simulink model "chap04_46"  (R2021a)
settings: Solver=FixedStepDiscrete  StartTime=0.0  StopTime=30  FixedStep=0.001  RelTol=1e-3
undefined symbols (not defined in the file): DiscIntNeverNeededParam
libraries: simulink x4
(part 1 of 4)
settings Model: Creator=陈天兴  LastModifiedBy=陈天兴

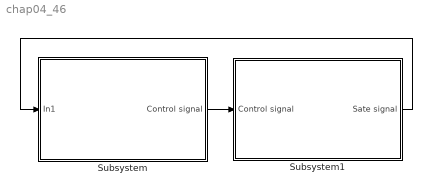
== system chap04_46 ==
  Subsystem : Subsystem
  Subsystem1 : Subsystem
  wires:
  Subsystem/1(Control signal) -> Subsystem1/1(Control signal)
  Subsystem1/1(Sate signal) -> Subsystem/1(In1)

== system chap04_46/Subsystem ==
  In1 : Inport
  Bus Creator : BusCreator  Inputs=6
  Bus Creator2 : BusCreator  Inputs=2
  Subsystem : Subsystem
  Subsystem1 : Subsystem
  Subsystem2 : Subsystem
  Subsystem3 : Subsystem
  Subsystem4 : Subsystem
  Subsystem5 : Subsystem
  Control signal : Outport
  wires:
  Bus Creator2/1 -> Subsystem/1(In19), Subsystem2/1(In19), Subsystem5/1(In19), Subsystem4/1(In19), Subsystem1/1(In19), Subsystem3/1(In19)
  Subsystem5/1(u3) -> Bus Creator/3
  Subsystem3/1(u4) -> Bus Creator/4
  Subsystem1/1(u5) -> Bus Creator/5
  Subsystem/1(u1) -> Bus Creator/1
  Subsystem2/1(u2) -> Bus Creator/2
  Subsystem4/1(u6) -> Bus Creator/6
  Bus Creator/1 -> [control], Control signal/1
  In1/1 -> Bus Creator2/1  "state(t)"
  [control] -> Bus Creator2/2  "control"

== system chap04_46/Subsystem1 ==
  Control signal : Inport
  Bus Creator : BusCreator  Inputs=7
  Bus Creator1 : BusCreator  Inputs=6
  Bus Selector : BusSelector  OutputSignals=node1.ux,node1.uy,node1.uz
  Bus Selector1 : BusSelector  OutputSignals=node2.ux,node2.uy,node2.uz
  Bus Selector2 : BusSelector  OutputSignals=node3.ux,node3.uy,node3.uz
  Bus Selector3 : BusSelector  OutputSignals=node4.ux,node4.uy,node4.uz
  Bus Selector4 : BusSelector  OutputSignals=node5.ux,node5.uy,node5.uz
  Bus Selector5 : BusSelector  OutputSignals=node6.ux,node6.uy,node6.uz
  Constant2 : Constant
  Scope : Scope  NumInputPorts=3
  Subsystem : Subsystem
  Subsystem1 : Subsystem
  Subsystem2 : Subsystem
  Subsystem3 : Subsystem
  Subsystem4 : Subsystem
  Subsystem5 : Subsystem
  Subsystem6 : Subsystem
  Subsystem7 : Subsystem
  Sate signal : Outport
  wires:
  Bus Creator/1 -> Sate signal/1
  Control signal/1 -> Bus Selector/1, Bus Selector1/1, Bus Selector5/1, Bus Selector4/1, Bus Selector3/1, Bus Selector2/1
  Bus Selector/1 -> Subsystem/4(ut1x)  "<ux>"
  Bus Selector/2 -> Subsystem/5(ut1y)  "<uy>"
  Bus Selector/3 -> Subsystem/6(ut1z)  "<uz>"
  Bus Selector1/1 -> Subsystem1/4(ut2x)  "<ux>"
  Bus Selector1/2 -> Subsystem1/5(ut2y)  "<uy>"
  Bus Selector1/3 -> Subsystem1/6(ut2z)  "<uz>"
  Bus Selector2/1 -> Subsystem2/4(ut3x)  "<ux>"
  Bus Selector2/2 -> Subsystem2/5(ut3y)  "<uy>"
  Bus Selector2/3 -> Subsystem2/6(ut3z)  "<uz>"
  Bus Selector3/1 -> Subsystem3/4(ut4x)  "<ux>"
  Bus Selector3/2 -> Subsystem3/5(ut4y)  "<uy>"
  Bus Selector3/3 -> Subsystem3/6(ut4z)  "<uz>"
  Bus Selector4/1 -> Subsystem4/4(ut5x)  "<ux>"
  Bus Selector4/2 -> Subsystem4/5(ut5y)  "<uy>"
  Bus Selector4/3 -> Subsystem4/6(ut5z)  "<uz>"
  Bus Selector5/1 -> Subsystem5/4(ut6x)  "<ux>"
  Bus Selector5/2 -> Subsystem5/5(ut6y)  "<uy>"
  Bus Selector5/3 -> Subsystem5/6(ut6z)  "<uz>"
  Subsystem5/1(node6) -> Bus Creator/7
  Subsystem4/1(node5) -> Bus Creator/6
  Subsystem3/1(node4) -> Bus Creator/5
  Subsystem2/1(node3) -> Bus Creator/4
  Subsystem1/1(node2) -> Bus Creator/3
  Subsystem/1(node1) -> Bus Creator/2
  Subsystem6/5(vy) -> Bus Creator1/5  "vy"
  Subsystem6/2(xy) -> Bus Creator1/2  "xy"
  Subsystem6/3(xz) -> Bus Creator1/3  "xz"
  Subsystem6/4(vx) -> Bus Creator1/4  "vx"
  Subsystem6/6(vz) -> Bus Creator1/6  "vz"
  Bus Creator1/1 -> Bus Creator/1  "node0"
  Subsystem6/1(xx) -> Bus Creator1/1  "xx"
  Subsystem7/2(dy) -> Subsystem/2(dy), Subsystem5/2(dy), Subsystem4/2(dy), Subsystem3/2(dy), Subsystem2/2(dy), Subsystem1/2(dy), Scope/2  "dy"
  Subsystem7/3(dz) -> Subsystem5/3(dz), Subsystem4/3(dz), Subsystem3/3(dz), Subsystem2/3(dz), Subsystem1/3(dz), Subsystem/3(dz), Scope/3  "dz"
  Subsystem7/1(dx) -> Subsystem3/1(dx), Subsystem5/1(dx), Subsystem4/1(dx), Subsystem2/1(dx), Subsystem1/1(dx), Subsystem/1(dx), Scope/1  "dx"
  Constant2/1 -> Subsystem7/1(switch)

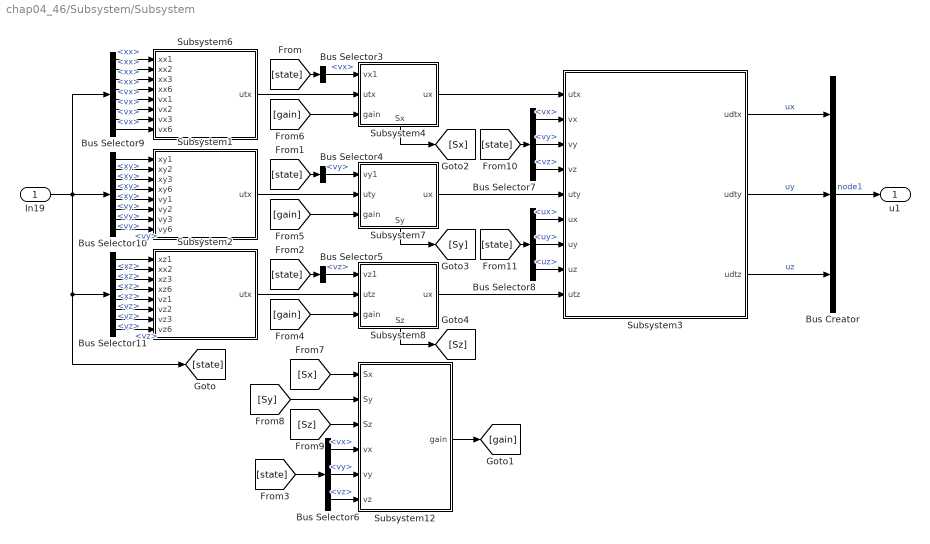
== system chap04_46/Subsystem/Subsystem ==
  In19 : Inport
  Bus Creator : BusCreator  Inputs=3
  Bus Selector10 : BusSelector  OutputSignals=state(t).node1.xy,state(t).node2.xy,state(t).node3.xy,state(t).node6.xy,state(t).node1.vy,state(t).node2.vy,state(t).node3.vy,state(t).node6.vy
  Bus Selector11 : BusSelector  OutputSignals=state(t).node1.xz,state(t).node2.xz,state(t).node3.xz,state(t).node6.xz,state(t).node1.vz,state(t).node2.vz,state(t).node3.vz,state(t).node6.vz
  Bus Selector3 : BusSelector  OutputSignals=state(t).node1.vx
  Bus Selector4 : BusSelector  OutputSignals=state(t).node1.vy
  Bus Selector5 : BusSelector  OutputSignals=state(t).node1.vz
  Bus Selector6 : BusSelector  OutputSignals=state(t).node1.vx,state(t).node1.vy,state(t).node1.vz
  Bus Selector7 : BusSelector  OutputSignals=state(t).node1.vx,state(t).node1.vy,state(t).node1.vz
  Bus Selector8 : BusSelector  OutputSignals=control.node1.ux,control.node1.uy,control.node1.uz
  Bus Selector9 : BusSelector  OutputSignals=state(t).node1.xx,state(t).node2.xx,state(t).node3.xx,state(t).node6.xx,state(t).node1.vx,state(t).node2.vx,state(t).node3.vx,state(t).node6.vx
  Subsystem1 : Subsystem
  Subsystem12 : Subsystem
  Subsystem2 : Subsystem
  Subsystem3 : Subsystem
  Subsystem4 : Subsystem
      settings: PortSchema="{\"entries\":[{\"content\":{\"sides\":[{\"content\":{\"connectorIds\":[\"In1\",\"In2\",\"In3\"]},\"type\":\"ConnectorPlacement.EquallySpacedRectSide\",\"uuid\":\"3c32f130-2df4-4697-80e9-267a8217898e\"},{\"content\":{\"connectorIds\":[\"Out1\"],\"side\":\"RIGHT\"},\"type\":\"ConnectorPlacement.EquallySpacedRectSide\",\"uuid\":\"840675a7-4714-440f-a6ce-75eff1b2763f\"},{\"content\":{\"connectorIds\":[],\"side\":\"TOP\"},\"type\":\"ConnectorPlacement.EquallySpacedRectSide\",\"uuid\":\"5c23af56-4ec3-4a39-a531-12998a0be3c8\"},{\"content\":{\"connectorIds\":[\"Out2\"],\"side\":\"BOTTOM\"},\"type\":\"ConnectorPlacement.EquallySpacedRectSide\",\"uuid\":\"31d953fb-65a0-42e9-a844-060de010f298\"}]},\"type\":\"ConnectorPlacement.EquallySpacedConnector\",\"uuid\":\"61b27aa3-5880-401e-bae3-4611093a191a\"}],\"packageUris\":[\"http://schema.mathworks.com/mf0/Connector/R2020b\"],\"version\":\"1.0\"}"
  Subsystem6 : Subsystem
  Subsystem7 : Subsystem
      settings: PortSchema="{\"entries\":[{\"content\":{\"sides\":[{\"content\":{\"connectorIds\":[\"In1\",\"In2\",\"In3\"]},\"type\":\"ConnectorPlacement.EquallySpacedRectSide\",\"uuid\":\"3c32f130-2df4-4697-80e9-267a8217898e\"},{\"content\":{\"connectorIds\":[\"Out1\"],\"side\":\"RIGHT\"},\"type\":\"ConnectorPlacement.EquallySpacedRectSide\",\"uuid\":\"840675a7-4714-440f-a6ce-75eff1b2763f\"},{\"content\":{\"connectorIds\":[],\"side\":\"TOP\"},\"type\":\"ConnectorPlacement.EquallySpacedRectSide\",\"uuid\":\"5c23af56-4ec3-4a39-a531-12998a0be3c8\"},{\"content\":{\"connectorIds\":[\"Out2\"],\"side\":\"BOTTOM\"},\"type\":\"ConnectorPlacement.EquallySpacedRectSide\",\"uuid\":\"31d953fb-65a0-42e9-a844-060de010f298\"}]},\"type\":\"ConnectorPlacement.EquallySpacedConnector\",\"uuid\":\"61b27aa3-5880-401e-bae3-4611093a191a\"}],\"packageUris\":[\"http://schema.mathworks.com/mf0/Connector/R2020b\"],\"version\":\"1.0\"}"
  Subsystem8 : Subsystem
      settings: PortSchema="{\"entries\":[{\"content\":{\"sides\":[{\"content\":{\"connectorIds\":[\"In1\",\"In2\",\"In3\"]},\"type\":\"ConnectorPlacement.EquallySpacedRectSide\",\"uuid\":\"3c32f130-2df4-4697-80e9-267a8217898e\"},{\"content\":{\"connectorIds\":[\"Out1\"],\"side\":\"RIGHT\"},\"type\":\"ConnectorPlacement.EquallySpacedRectSide\",\"uuid\":\"840675a7-4714-440f-a6ce-75eff1b2763f\"},{\"content\":{\"connectorIds\":[],\"side\":\"TOP\"},\"type\":\"ConnectorPlacement.EquallySpacedRectSide\",\"uuid\":\"5c23af56-4ec3-4a39-a531-12998a0be3c8\"},{\"content\":{\"connectorIds\":[\"Out2\"],\"side\":\"BOTTOM\"},\"type\":\"ConnectorPlacement.EquallySpacedRectSide\",\"uuid\":\"31d953fb-65a0-42e9-a844-060de010f298\"}]},\"type\":\"ConnectorPlacement.EquallySpacedConnector\",\"uuid\":\"61b27aa3-5880-401e-bae3-4611093a191a\"}],\"packageUris\":[\"http://schema.mathworks.com/mf0/Connector/R2020b\"],\"version\":\"1.0\"}"
  u1 : Outport
  wires:
  Subsystem2/1(utx) -> Subsystem8/2(utz)
  Subsystem6/1(utx) -> Subsystem4/2(utx)
  Subsystem1/1(utx) -> Subsystem7/2(uty)
  Bus Creator/1 -> u1/1  "node1"
  In19/1 -> Bus Selector10/1, Bus Selector9/1, Bus Selector11/1, [state]
  Bus Selector9/1 -> Subsystem6/1(xx1)  "<xx>"
  Bus Selector9/2 -> Subsystem6/2(xx2)  "<xx>"
  Bus Selector9/3 -> Subsystem6/3(xx3)  "<xx>"
  Bus Selector9/4 -> Subsystem6/4(xx6)  "<xx>"
  Bus Selector9/5 -> Subsystem6/5(vx1)  "<vx>"
  Bus Selector9/6 -> Subsystem6/6(vx2)  "<vx>"
  Bus Selector9/7 -> Subsystem6/7(vx3)  "<vx>"
  Bus Selector9/8 -> Subsystem6/8(vx6)  "<vx>"
  Bus Selector10/1 -> Subsystem1/1(xy1)  "<xy>"
  Bus Selector10/2 -> Subsystem1/2(xy2)  "<xy>"
  Bus Selector10/3 -> Subsystem1/3(xy3)  "<xy>"
  Bus Selector10/4 -> Subsystem1/4(xy6)  "<xy>"
  Bus Selector10/5 -> Subsystem1/5(vy1)  "<vy>"
  Bus Selector10/6 -> Subsystem1/6(vy2)  "<vy>"
  Bus Selector10/7 -> Subsystem1/7(vy3)  "<vy>"
  Bus Selector10/8 -> Subsystem1/8(vy6)  "<vy>"
  Bus Selector11/1 -> Subsystem2/1(xz1)  "<xz>"
  Bus Selector11/2 -> Subsystem2/2(xx2)  "<xz>"
  Bus Selector11/3 -> Subsystem2/3(xz3)  "<xz>"
  Bus Selector11/4 -> Subsystem2/4(xz6)  "<xz>"
  Bus Selector11/5 -> Subsystem2/5(vz1)  "<vz>"
  Bus Selector11/6 -> Subsystem2/6(vz2)  "<vz>"
  Bus Selector11/7 -> Subsystem2/7(vz3)  "<vz>"
  Bus Selector11/8 -> Subsystem2/8(vz6)  "<vz>"
  [state] -> Bus Selector3/1
  Bus Selector3/1 -> Subsystem4/1(vx1)  "<vx>"
  Bus Selector4/1 -> Subsystem7/1(vy1)  "<vy>"
  [state] -> Bus Selector4/1
  [state] -> Bus Selector5/1
  Bus Selector5/1 -> Subsystem8/1(vz1)  "<vz>"
  [state] -> Bus Selector6/1
  Bus Selector6/2 -> Subsystem12/5(vy)  "<vy>"
  Bus Selector6/1 -> Subsystem12/4(vx)  "<vx>"
  Bus Selector6/3 -> Subsystem12/6(vz)  "<vz>"
  Subsystem12/1(" gain") -> [gain]
  [gain] -> Subsystem8/3(gain)
  [gain] -> Subsystem7/3(gain)
  [gain] -> Subsystem4/3(gain)
  Subsystem4/2(Sx) -> [Sx]
  Subsystem7/2(Sy) -> [Sy]
  Subsystem8/2(Sz) -> [Sz]
  [Sx] -> Subsystem12/1(Sx)
  [Sy] -> Subsystem12/2(Sy)
  [Sz] -> Subsystem12/3(Sz)
  Subsystem3/1(udtx) -> Bus Creator/1  "ux"
  Subsystem3/2(udty) -> Bus Creator/2  "uy"
  Subsystem3/3(udtz) -> Bus Creator/3  "uz"
  Subsystem4/1(ux) -> Subsystem3/1(utx)
  Subsystem7/1(ux) -> Subsystem3/5(uty)
  Subsystem8/1(ux) -> Subsystem3/9(utz)
  [state] -> Bus Selector7/1
  Bus Selector7/1 -> Subsystem3/2(vx)  "<vx>"
  Bus Selector7/2 -> Subsystem3/3(vy)  "<vy>"
  Bus Selector7/3 -> Subsystem3/4(vz)  "<vz>"
  [state] -> Bus Selector8/1
  Bus Selector8/1 -> Subsystem3/6(ux)  "<ux>"
  Bus Selector8/2 -> Subsystem3/7(uy)  "<uy>"
  Bus Selector8/3 -> Subsystem3/8(uz)  "<uz>"

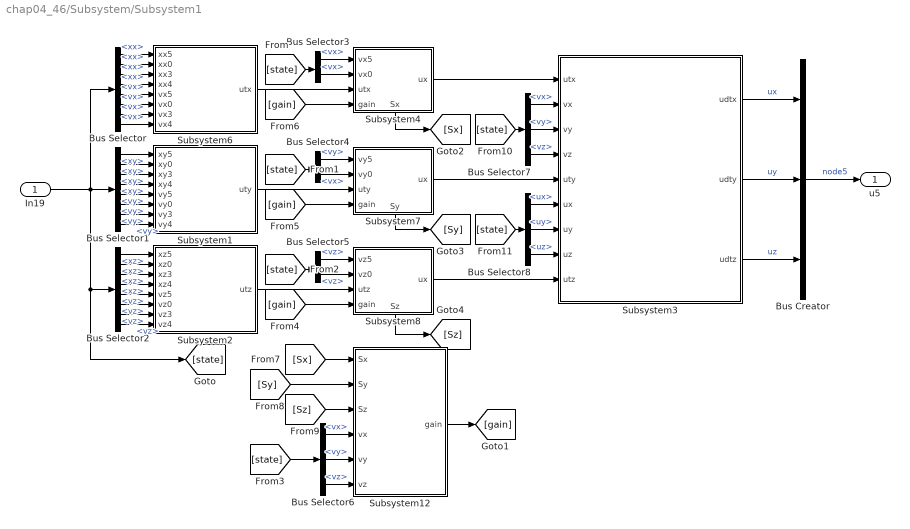
== system chap04_46/Subsystem/Subsystem1 ==
  In19 : Inport
  Bus Creator : BusCreator  Inputs=3
  Bus Selector : BusSelector  OutputSignals=state(t).node5.xx,state(t).node0.xx,state(t).node3.xx,state(t).node4.xx,state(t).node5.vx,state(t).node0.vx,state(t).node3.vx,state(t).node4.vx
  Bus Selector1 : BusSelector  OutputSignals=state(t).node5.xy,state(t).node0.xy,state(t).node3.xy,state(t).node4.xy,state(t).node5.vy,state(t).node0.vy,state(t).node3.vy,state(t).node4.vy
  Bus Selector2 : BusSelector  OutputSignals=state(t).node5.xz,state(t).node0.xz,state(t).node3.xz,state(t).node4.xz,state(t).node5.vz,state(t).node0.vz,state(t).node3.vz,state(t).node4.vz
  Bus Selector3 : BusSelector  OutputSignals=state(t).node5.vx,state(t).node0.vx
  Bus Selector4 : BusSelector  OutputSignals=state(t).node5.vy,state(t).node0.vx
  Bus Selector5 : BusSelector  OutputSignals=state(t).node5.vz,state(t).node0.vz
  Bus Selector6 : BusSelector  OutputSignals=state(t).node5.vx,state(t).node5.vy,state(t).node5.vz
  Bus Selector7 : BusSelector  OutputSignals=state(t).node5.vx,state(t).node5.vy,state(t).node5.vz
  Bus Selector8 : BusSelector  OutputSignals=control.node5.ux,control.node5.uy,control.node5.uz
  Subsystem1 : Subsystem
  Subsystem12 : Subsystem
  Subsystem2 : Subsystem
  Subsystem3 : Subsystem
  Subsystem4 : Subsystem
      settings: PortSchema="{\"entries\":[{\"content\":{\"sides\":[{\"content\":{\"connectorIds\":[\"In1\",\"In2\",\"In3\",\"In4\"]},\"type\":\"ConnectorPlacement.EquallySpacedRectSide\",\"uuid\":\"3c32f130-2df4-4697-80e9-267a8217898e\"},{\"content\":{\"connectorIds\":[\"Out1\"],\"side\":\"RIGHT\"},\"type\":\"ConnectorPlacement.EquallySpacedRectSide\",\"uuid\":\"840675a7-4714-440f-a6ce-75eff1b2763f\"},{\"content\":{\"connectorIds\":[],\"side\":\"TOP\"},\"type\":\"ConnectorPlacement.EquallySpacedRectSide\",\"uuid\":\"5c23af56-4ec3-4a39-a531-12998a0be3c8\"},{\"content\":{\"connectorIds\":[\"Out2\"],\"side\":\"BOTTOM\"},\"type\":\"ConnectorPlacement.EquallySpacedRectSide\",\"uuid\":\"31d953fb-65a0-42e9-a844-060de010f298\"}]},\"type\":\"ConnectorPlacement.EquallySpacedConnector\",\"uuid\":\"61b27aa3-5880-401e-bae3-4611093a191a\"}],\"packageUris\":[\"http://schema.mathworks.com/mf0/Connector/R2020b\"],\"version\":\"1.0\"}"
  Subsystem6 : Subsystem
  Subsystem7 : Subsystem
      settings: PortSchema="{\"entries\":[{\"content\":{\"sides\":[{\"content\":{\"connectorIds\":[\"In1\",\"In2\",\"In3\",\"In4\"]},\"type\":\"ConnectorPlacement.EquallySpacedRectSide\",\"uuid\":\"3c32f130-2df4-4697-80e9-267a8217898e\"},{\"content\":{\"connectorIds\":[\"Out1\"],\"side\":\"RIGHT\"},\"type\":\"ConnectorPlacement.EquallySpacedRectSide\",\"uuid\":\"840675a7-4714-440f-a6ce-75eff1b2763f\"},{\"content\":{\"connectorIds\":[],\"side\":\"TOP\"},\"type\":\"ConnectorPlacement.EquallySpacedRectSide\",\"uuid\":\"5c23af56-4ec3-4a39-a531-12998a0be3c8\"},{\"content\":{\"connectorIds\":[\"Out2\"],\"side\":\"BOTTOM\"},\"type\":\"ConnectorPlacement.EquallySpacedRectSide\",\"uuid\":\"31d953fb-65a0-42e9-a844-060de010f298\"}]},\"type\":\"ConnectorPlacement.EquallySpacedConnector\",\"uuid\":\"61b27aa3-5880-401e-bae3-4611093a191a\"}],\"packageUris\":[\"http://schema.mathworks.com/mf0/Connector/R2020b\"],\"version\":\"1.0\"}"
  Subsystem8 : Subsystem
      settings: PortSchema="{\"entries\":[{\"content\":{\"sides\":[{\"content\":{\"connectorIds\":[\"In1\",\"In2\",\"In3\",\"In4\"]},\"type\":\"ConnectorPlacement.EquallySpacedRectSide\",\"uuid\":\"3c32f130-2df4-4697-80e9-267a8217898e\"},{\"content\":{\"connectorIds\":[\"Out1\"],\"side\":\"RIGHT\"},\"type\":\"ConnectorPlacement.EquallySpacedRectSide\",\"uuid\":\"840675a7-4714-440f-a6ce-75eff1b2763f\"},{\"content\":{\"connectorIds\":[],\"side\":\"TOP\"},\"type\":\"ConnectorPlacement.EquallySpacedRectSide\",\"uuid\":\"5c23af56-4ec3-4a39-a531-12998a0be3c8\"},{\"content\":{\"connectorIds\":[\"Out2\"],\"side\":\"BOTTOM\"},\"type\":\"ConnectorPlacement.EquallySpacedRectSide\",\"uuid\":\"31d953fb-65a0-42e9-a844-060de010f298\"}]},\"type\":\"ConnectorPlacement.EquallySpacedConnector\",\"uuid\":\"61b27aa3-5880-401e-bae3-4611093a191a\"}],\"packageUris\":[\"http://schema.mathworks.com/mf0/Connector/R2020b\"],\"version\":\"1.0\"}"
  u5 : Outport
  wires:
  Bus Creator/1 -> u5/1  "node5"
  Bus Selector/5 -> Subsystem6/5(vx5)  "<vx>"
  Bus Selector/1 -> Subsystem6/1(xx5)  "<xx>"
  Bus Selector/3 -> Subsystem6/3(xx3)  "<xx>"
  Bus Selector/8 -> Subsystem6/8(vx4)  "<vx>"
  Bus Selector/7 -> Subsystem6/7(vx3)  "<vx>"
  Bus Selector/4 -> Subsystem6/4(xx4)  "<xx>"
  Bus Selector6/3 -> Subsystem12/6(vz)  "<vz>"
  Bus Selector6/1 -> Subsystem12/4(vx)  "<vx>"
  [Sx] -> Subsystem12/1(Sx)
  [Sz] -> Subsystem12/3(Sz)
  Subsystem12/1(" gain") -> [gain]
  In19/1 -> Bus Selector/1, Bus Selector1/1, Bus Selector2/1, [state]
  [state] -> Bus Selector6/1
  [Sy] -> Subsystem12/2(Sy)
  Bus Selector6/2 -> Subsystem12/5(vy)  "<vy>"
  Subsystem3/3(udtz) -> Bus Creator/3  "uz"
  Subsystem3/2(udty) -> Bus Creator/2  "uy"
  Subsystem3/1(udtx) -> Bus Creator/1  "ux"
  [state] -> Bus Selector7/1
  Bus Selector8/1 -> Subsystem3/6(ux)  "<ux>"
  Bus Selector7/2 -> Subsystem3/3(vy)  "<vy>"
  Bus Selector8/2 -> Subsystem3/7(uy)  "<uy>"
  [state] -> Bus Selector8/1
  Bus Selector7/1 -> Subsystem3/2(vx)  "<vx>"
  Bus Selector7/3 -> Subsystem3/4(vz)  "<vz>"
  Bus Selector8/3 -> Subsystem3/8(uz)  "<uz>"
  Bus Selector/2 -> Subsystem6/2(xx0)  "<xx>"
  Bus Selector/6 -> Subsystem6/6(vx0)  "<vx>"
  Bus Selector1/1 -> Subsystem1/1(xy5)  "<xy>"
  Bus Selector1/2 -> Subsystem1/2(xy0)  "<xy>"
  Bus Selector1/3 -> Subsystem1/3(xy3)  "<xy>"
  Bus Selector1/4 -> Subsystem1/4(xy4)  "<xy>"
  Bus Selector1/5 -> Subsystem1/5(vy5)  "<vy>"
  Bus Selector1/6 -> Subsystem1/6(vy0)  "<vy>"
  Bus Selector1/7 -> Subsystem1/7(vy3)  "<vy>"
  Bus Selector1/8 -> Subsystem1/8(vy4)  "<vy>"
  Bus Selector2/1 -> Subsystem2/1(xz5)  "<xz>"
  Bus Selector2/2 -> Subsystem2/2(xz0)  "<xz>"
  Bus Selector2/3 -> Subsystem2/3(xz3)  "<xz>"
  Bus Selector2/4 -> Subsystem2/4(xz4)  "<xz>"
  Bus Selector2/5 -> Subsystem2/5(vz5)  "<vz>"
  Bus Selector2/6 -> Subsystem2/6(vz0)  "<vz>"
  Bus Selector2/7 -> Subsystem2/7(vz3)  "<vz>"
  Bus Selector2/8 -> Subsystem2/8(vz4)  "<vz>"
  [gain] -> Subsystem8/4(gain)
  Subsystem7/1(ux) -> Subsystem3/5(uty)
  Subsystem2/1(utz) -> Subsystem8/3(utz)
  Subsystem1/1(uty) -> Subsystem7/3(uty)
  [state] -> Bus Selector3/1
  Subsystem4/1(ux) -> Subsystem3/1(utx)
  Bus Selector3/2 -> Subsystem4/2(vx0)  "<vx>"
  Bus Selector3/1 -> Subsystem4/1(vx5)  "<vx>"
  Subsystem8/1(ux) -> Subsystem3/9(utz)
  Bus Selector5/1 -> Subsystem8/1(vz5)  "<vz>"
  [state] -> Bus Selector4/1
  Subsystem6/1(utx) -> Subsystem4/3(utx)
  [state] -> Bus Selector5/1
  Bus Selector4/1 -> Subsystem7/1(vy5)  "<vy>"
  Bus Selector4/2 -> Subsystem7/2(vy0)  "<vx>"
  Bus Selector5/2 -> Subsystem8/2(vz0)  "<vz>"
  [gain] -> Subsystem4/4(gain)
  Subsystem4/2(Sx) -> [Sx]
  Subsystem7/2(Sy) -> [Sy]
  Subsystem8/2(Sz) -> [Sz]
  [gain] -> Subsystem7/4(gain)

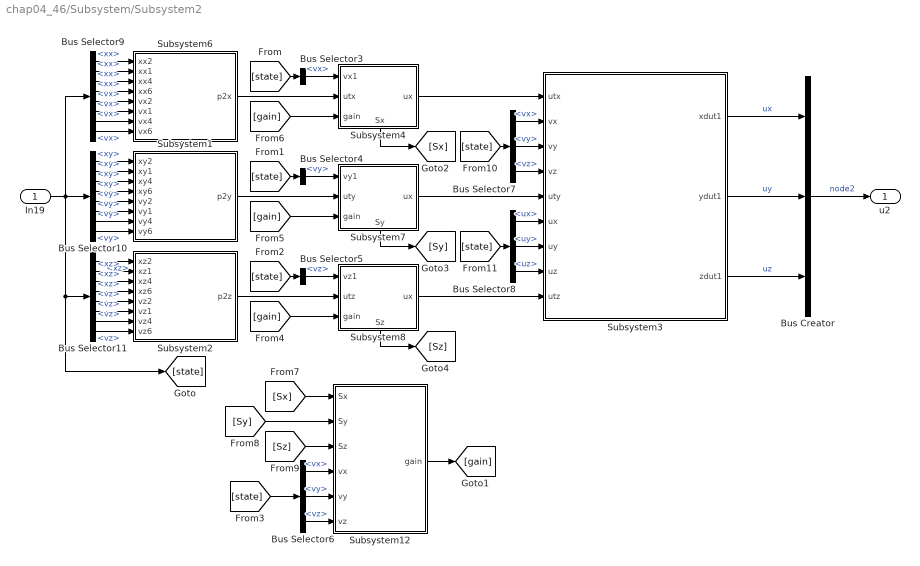
== system chap04_46/Subsystem/Subsystem2 ==
  In19 : Inport
  Bus Creator : BusCreator  Inputs=3
  Bus Selector10 : BusSelector  OutputSignals=state(t).node2.xy,state(t).node1.xy,state(t).node4.xy,state(t).node6.xy,state(t).node2.vy,state(t).node1.vy,state(t).node4.vy,state(t).node6.vy
  Bus Selector11 : BusSelector  OutputSignals=state(t).node2.xz,state(t).node1.xz,state(t).node4.xz,state(t).node6.xz,state(t).node2.vz,state(t).node1.vz,state(t).node4.vz,state(t).node6.vz
  Bus Selector3 : BusSelector  OutputSignals=state(t).node2.vx
  Bus Selector4 : BusSelector  OutputSignals=state(t).node2.vy
  Bus Selector5 : BusSelector  OutputSignals=state(t).node2.vz
  Bus Selector6 : BusSelector  OutputSignals=state(t).node2.vx,state(t).node2.vy,state(t).node2.vz
  Bus Selector7 : BusSelector  OutputSignals=state(t).node2.vx,state(t).node2.vy,state(t).node2.vz
  Bus Selector8 : BusSelector  OutputSignals=control.node2.ux,control.node2.uy,control.node2.uz
  Bus Selector9 : BusSelector  OutputSignals=state(t).node2.xx,state(t).node1.xx,state(t).node4.xx,state(t).node6.xx,state(t).node2.vx,state(t).node1.vx,state(t).node4.vx,state(t).node6.vx
  Subsystem1 : Subsystem
  Subsystem12 : Subsystem
  Subsystem2 : Subsystem
  Subsystem3 : Subsystem
  Subsystem4 : Subsystem
      settings: PortSchema="{\"entries\":[{\"content\":{\"sides\":[{\"content\":{\"connectorIds\":[\"In1\",\"In2\",\"In3\"]},\"type\":\"ConnectorPlacement.EquallySpacedRectSide\",\"uuid\":\"3c32f130-2df4-4697-80e9-267a8217898e\"},{\"content\":{\"connectorIds\":[\"Out1\"],\"side\":\"RIGHT\"},\"type\":\"ConnectorPlacement.EquallySpacedRectSide\",\"uuid\":\"840675a7-4714-440f-a6ce-75eff1b2763f\"},{\"content\":{\"connectorIds\":[],\"side\":\"TOP\"},\"type\":\"ConnectorPlacement.EquallySpacedRectSide\",\"uuid\":\"5c23af56-4ec3-4a39-a531-12998a0be3c8\"},{\"content\":{\"connectorIds\":[\"Out2\"],\"side\":\"BOTTOM\"},\"type\":\"ConnectorPlacement.EquallySpacedRectSide\",\"uuid\":\"31d953fb-65a0-42e9-a844-060de010f298\"}]},\"type\":\"ConnectorPlacement.EquallySpacedConnector\",\"uuid\":\"61b27aa3-5880-401e-bae3-4611093a191a\"}],\"packageUris\":[\"http://schema.mathworks.com/mf0/Connector/R2020b\"],\"version\":\"1.0\"}"
  Subsystem6 : Subsystem
  Subsystem7 : Subsystem
      settings: PortSchema="{\"entries\":[{\"content\":{\"sides\":[{\"content\":{\"connectorIds\":[\"In1\",\"In2\",\"In3\"]},\"type\":\"ConnectorPlacement.EquallySpacedRectSide\",\"uuid\":\"3c32f130-2df4-4697-80e9-267a8217898e\"},{\"content\":{\"connectorIds\":[\"Out1\"],\"side\":\"RIGHT\"},\"type\":\"ConnectorPlacement.EquallySpacedRectSide\",\"uuid\":\"840675a7-4714-440f-a6ce-75eff1b2763f\"},{\"content\":{\"connectorIds\":[],\"side\":\"TOP\"},\"type\":\"ConnectorPlacement.EquallySpacedRectSide\",\"uuid\":\"5c23af56-4ec3-4a39-a531-12998a0be3c8\"},{\"content\":{\"connectorIds\":[\"Out2\"],\"side\":\"BOTTOM\"},\"type\":\"ConnectorPlacement.EquallySpacedRectSide\",\"uuid\":\"31d953fb-65a0-42e9-a844-060de010f298\"}]},\"type\":\"ConnectorPlacement.EquallySpacedConnector\",\"uuid\":\"61b27aa3-5880-401e-bae3-4611093a191a\"}],\"packageUris\":[\"http://schema.mathworks.com/mf0/Connector/R2020b\"],\"version\":\"1.0\"}"
  Subsystem8 : Subsystem
      settings: PortSchema="{\"entries\":[{\"content\":{\"sides\":[{\"content\":{\"connectorIds\":[\"In1\",\"In2\",\"In3\"]},\"type\":\"ConnectorPlacement.EquallySpacedRectSide\",\"uuid\":\"3c32f130-2df4-4697-80e9-267a8217898e\"},{\"content\":{\"connectorIds\":[\"Out1\"],\"side\":\"RIGHT\"},\"type\":\"ConnectorPlacement.EquallySpacedRectSide\",\"uuid\":\"840675a7-4714-440f-a6ce-75eff1b2763f\"},{\"content\":{\"connectorIds\":[],\"side\":\"TOP\"},\"type\":\"ConnectorPlacement.EquallySpacedRectSide\",\"uuid\":\"5c23af56-4ec3-4a39-a531-12998a0be3c8\"},{\"content\":{\"connectorIds\":[\"Out2\"],\"side\":\"BOTTOM\"},\"type\":\"ConnectorPlacement.EquallySpacedRectSide\",\"uuid\":\"31d953fb-65a0-42e9-a844-060de010f298\"}]},\"type\":\"ConnectorPlacement.EquallySpacedConnector\",\"uuid\":\"61b27aa3-5880-401e-bae3-4611093a191a\"}],\"packageUris\":[\"http://schema.mathworks.com/mf0/Connector/R2020b\"],\"version\":\"1.0\"}"
  u2 : Outport
  wires:
  Bus Creator/1 -> u2/1  "node2"
  Bus Selector6/1 -> Subsystem12/4(vx)  "<vx>"
  Bus Selector6/2 -> Subsystem12/5(vy)  "<vy>"
  Bus Selector6/3 -> Subsystem12/6(vz)  "<vz>"
  [Sz] -> Subsystem12/3(Sz)
  [Sx] -> Subsystem12/1(Sx)
  [state] -> Bus Selector6/1
  [Sy] -> Subsystem12/2(Sy)
  Subsystem12/1(" gain") -> [gain]
  Subsystem3/1(xdut1) -> Bus Creator/1  "ux"
  Subsystem3/2(ydut1) -> Bus Creator/2  "uy"
  Subsystem3/3(zdut1) -> Bus Creator/3  "uz"
  Bus Selector8/3 -> Subsystem3/8(uz)  "<uz>"
  Bus Selector7/3 -> Subsystem3/4(vz)  "<vz>"
  Bus Selector7/2 -> Subsystem3/3(vy)  "<vy>"
  Bus Selector7/1 -> Subsystem3/2(vx)  "<vx>"
  Bus Selector8/1 -> Subsystem3/6(ux)  "<ux>"
  [state] -> Bus Selector7/1
  Bus Selector8/2 -> Subsystem3/7(uy)  "<uy>"
  [state] -> Bus Selector8/1
  Subsystem8/2(Sz) -> [Sz]
  Subsystem7/1(ux) -> Subsystem3/5(uty)
  Subsystem1/1(p2y) -> Subsystem7/2(uty)
  [state] -> Bus Selector4/1
  Subsystem4/1(ux) -> Subsystem3/1(utx)
  Subsystem2/1(p2z) -> Subsystem8/2(utz)
  Bus Selector4/1 -> Subsystem7/1(vy1)  "<vy>"
  Bus Selector5/1 -> Subsystem8/1(vz1)  "<vz>"
  [gain] -> Subsystem8/3(gain)
  [gain] -> Subsystem4/3(gain)
  Subsystem8/1(ux) -> Subsystem3/9(utz)
  [gain] -> Subsystem7/3(gain)
  [state] -> Bus Selector3/1
  Subsystem6/1(p2x) -> Subsystem4/2(utx)
  Subsystem7/2(Sy) -> [Sy]
  Bus Selector3/1 -> Subsystem4/1(vx1)  "<vx>"
  Subsystem4/2(Sx) -> [Sx]
  [state] -> Bus Selector5/1
  In19/1 -> Bus Selector9/1, Bus Selector10/1, Bus Selector11/1, [state]
  Bus Selector10/6 -> Subsystem1/6(vy1)  "<vy>"
  Bus Selector11/6 -> Subsystem2/6(vz1)  "<vz>"
  Bus Selector9/7 -> Subsystem6/7(vx4)  "<vx>"
  Bus Selector9/3 -> Subsystem6/3(xx4)  "<xx>"
  Bus Selector10/2 -> Subsystem1/2(xy1)  "<xy>"
  Bus Selector10/5 -> Subsystem1/5(vy2)  "<vy>"
  Bus Selector9/2 -> Subsystem6/2(xx1)  "<xx>"
  Bus Selector9/6 -> Subsystem6/6(vx1)  "<vx>"
  Bus Selector9/8 -> Subsystem6/8(vx6)  "<vx>"
  Bus Selector10/8 -> Subsystem1/8(vy6)  "<vy>"
  Bus Selector9/1 -> Subsystem6/1(xx2)  "<xx>"
  Bus Selector9/5 -> Subsystem6/5(vx2)  "<vx>"
  Bus Selector10/1 -> Subsystem1/1(xy2)  "<xy>"
  Bus Selector11/3 -> Subsystem2/3(xz4)  "<xz>"
  Bus Selector11/4 -> Subsystem2/4(xz6)  "<xz>"
  Bus Selector11/5 -> Subsystem2/5(vz2)  "<vz>"
  Bus Selector11/7 -> Subsystem2/7(vz4)  "<vz>"
  Bus Selector11/1 -> Subsystem2/1(xz2)  "<xz>"
  Bus Selector11/2 -> Subsystem2/2(xz1)  "<xz>"
  Bus Selector10/7 -> Subsystem1/7(vy4)  "<vy>"
  Bus Selector10/3 -> Subsystem1/3(xy4)  "<xy>"
  Bus Selector10/4 -> Subsystem1/4(xy6)  "<xy>"
  Bus Selector9/4 -> Subsystem6/4(xx6)  "<xx>"
  Bus Selector11/8 -> Subsystem2/8(vz6)  "<vz>"

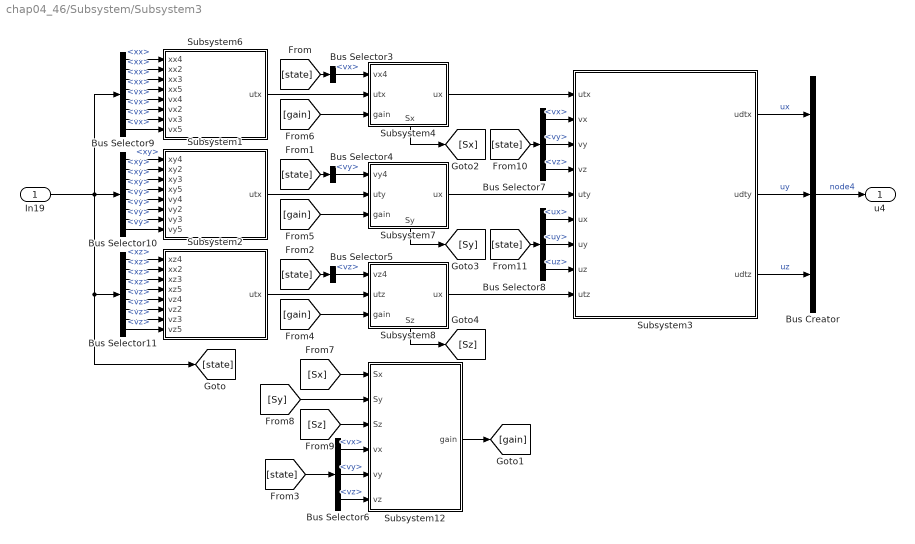
== system chap04_46/Subsystem/Subsystem3 ==
  In19 : Inport
  Bus Creator : BusCreator  Inputs=3
  Bus Selector10 : BusSelector  OutputSignals=state(t).node4.xy,state(t).node2.xy,state(t).node3.xy,state(t).node5.xy,state(t).node4.vy,state(t).node2.vy,state(t).node3.vy,state(t).node5.vy
  Bus Selector11 : BusSelector  OutputSignals=state(t).node4.xz,state(t).node2.xz,state(t).node3.xz,state(t).node5.xz,state(t).node4.vz,state(t).node2.vz,state(t).node3.vz,state(t).node5.vz
  Bus Selector3 : BusSelector  OutputSignals=state(t).node4.vx
  Bus Selector4 : BusSelector  OutputSignals=state(t).node4.vy
  Bus Selector5 : BusSelector  OutputSignals=state(t).node4.vz
  Bus Selector6 : BusSelector  OutputSignals=state(t).node4.vx,state(t).node4.vy,state(t).node4.vz
  Bus Selector7 : BusSelector  OutputSignals=state(t).node4.vx,state(t).node4.vy,state(t).node4.vz
  Bus Selector8 : BusSelector  OutputSignals=control.node4.ux,control.node4.uy,control.node4.uz
  Bus Selector9 : BusSelector  OutputSignals=state(t).node4.xx,state(t).node2.xx,state(t).node3.xx,state(t).node5.xx,state(t).node4.vx,state(t).node2.vx,state(t).node3.vx,state(t).node5.vx
  Subsystem1 : Subsystem
  Subsystem12 : Subsystem
  Subsystem2 : Subsystem
  Subsystem3 : Subsystem
  Subsystem4 : Subsystem
      settings: PortSchema="{\"entries\":[{\"content\":{\"sides\":[{\"content\":{\"connectorIds\":[\"In1\",\"In2\",\"In3\"]},\"type\":\"ConnectorPlacement.EquallySpacedRectSide\",\"uuid\":\"3c32f130-2df4-4697-80e9-267a8217898e\"},{\"content\":{\"connectorIds\":[\"Out1\"],\"side\":\"RIGHT\"},\"type\":\"ConnectorPlacement.EquallySpacedRectSide\",\"uuid\":\"840675a7-4714-440f-a6ce-75eff1b2763f\"},{\"content\":{\"connectorIds\":[],\"side\":\"TOP\"},\"type\":\"ConnectorPlacement.EquallySpacedRectSide\",\"uuid\":\"5c23af56-4ec3-4a39-a531-12998a0be3c8\"},{\"content\":{\"connectorIds\":[\"Out2\"],\"side\":\"BOTTOM\"},\"type\":\"ConnectorPlacement.EquallySpacedRectSide\",\"uuid\":\"31d953fb-65a0-42e9-a844-060de010f298\"}]},\"type\":\"ConnectorPlacement.EquallySpacedConnector\",\"uuid\":\"61b27aa3-5880-401e-bae3-4611093a191a\"}],\"packageUris\":[\"http://schema.mathworks.com/mf0/Connector/R2020b\"],\"version\":\"1.0\"}"
  Subsystem6 : Subsystem
  Subsystem7 : Subsystem
      settings: PortSchema="{\"entries\":[{\"content\":{\"sides\":[{\"content\":{\"connectorIds\":[\"In1\",\"In2\",\"In3\"]},\"type\":\"ConnectorPlacement.EquallySpacedRectSide\",\"uuid\":\"3c32f130-2df4-4697-80e9-267a8217898e\"},{\"content\":{\"connectorIds\":[\"Out1\"],\"side\":\"RIGHT\"},\"type\":\"ConnectorPlacement.EquallySpacedRectSide\",\"uuid\":\"840675a7-4714-440f-a6ce-75eff1b2763f\"},{\"content\":{\"connectorIds\":[],\"side\":\"TOP\"},\"type\":\"ConnectorPlacement.EquallySpacedRectSide\",\"uuid\":\"5c23af56-4ec3-4a39-a531-12998a0be3c8\"},{\"content\":{\"connectorIds\":[\"Out2\"],\"side\":\"BOTTOM\"},\"type\":\"ConnectorPlacement.EquallySpacedRectSide\",\"uuid\":\"31d953fb-65a0-42e9-a844-060de010f298\"}]},\"type\":\"ConnectorPlacement.EquallySpacedConnector\",\"uuid\":\"61b27aa3-5880-401e-bae3-4611093a191a\"}],\"packageUris\":[\"http://schema.mathworks.com/mf0/Connector/R2020b\"],\"version\":\"1.0\"}"
  Subsystem8 : Subsystem
      settings: PortSchema="{\"entries\":[{\"content\":{\"sides\":[{\"content\":{\"connectorIds\":[\"In1\",\"In2\",\"In3\"]},\"type\":\"ConnectorPlacement.EquallySpacedRectSide\",\"uuid\":\"3c32f130-2df4-4697-80e9-267a8217898e\"},{\"content\":{\"connectorIds\":[\"Out1\"],\"side\":\"RIGHT\"},\"type\":\"ConnectorPlacement.EquallySpacedRectSide\",\"uuid\":\"840675a7-4714-440f-a6ce-75eff1b2763f\"},{\"content\":{\"connectorIds\":[],\"side\":\"TOP\"},\"type\":\"ConnectorPlacement.EquallySpacedRectSide\",\"uuid\":\"5c23af56-4ec3-4a39-a531-12998a0be3c8\"},{\"content\":{\"connectorIds\":[\"Out2\"],\"side\":\"BOTTOM\"},\"type\":\"ConnectorPlacement.EquallySpacedRectSide\",\"uuid\":\"31d953fb-65a0-42e9-a844-060de010f298\"}]},\"type\":\"ConnectorPlacement.EquallySpacedConnector\",\"uuid\":\"61b27aa3-5880-401e-bae3-4611093a191a\"}],\"packageUris\":[\"http://schema.mathworks.com/mf0/Connector/R2020b\"],\"version\":\"1.0\"}"
  u4 : Outport
  wires:
  Bus Creator/1 -> u4/1  "node4"
  Bus Selector9/2 -> Subsystem6/2(xx2)  "<xx>"
  Bus Selector10/7 -> Subsystem1/7(vy3)  "<vy>"
  Bus Selector10/4 -> Subsystem1/4(xy5)  "<xy>"
  Bus Selector11/3 -> Subsystem2/3(xz3)  "<xz>"
  Bus Selector9/8 -> Subsystem6/8(vx5)  "<vx>"
  Bus Selector11/2 -> Subsystem2/2(xx2)  "<xz>"
  Bus Selector11/4 -> Subsystem2/4(xz5)  "<xz>"
  Bus Selector10/5 -> Subsystem1/5(vy4)  "<vy>"
  Bus Selector10/2 -> Subsystem1/2(xy2)  "<xy>"
  Bus Selector11/7 -> Subsystem2/7(vz3)  "<vz>"
  Bus Selector11/5 -> Subsystem2/5(vz4)  "<vz>"
  Bus Selector10/6 -> Subsystem1/6(vy2)  "<vy>"
  Bus Selector11/8 -> Subsystem2/8(vz5)  "<vz>"
  Bus Selector11/6 -> Subsystem2/6(vz2)  "<vz>"
  Bus Selector10/3 -> Subsystem1/3(xy3)  "<xy>"
  Bus Selector11/1 -> Subsystem2/1(xz4)  "<xz>"
  Bus Selector9/5 -> Subsystem6/5(vx4)  "<vx>"
  Bus Selector9/1 -> Subsystem6/1(xx4)  "<xx>"
  Bus Selector9/3 -> Subsystem6/3(xx3)  "<xx>"
  Bus Selector10/8 -> Subsystem1/8(vy5)  "<vy>"
  Bus Selector10/1 -> Subsystem1/1(xy4)  "<xy>"
  Bus Selector9/7 -> Subsystem6/7(vx3)  "<vx>"
  Bus Selector9/6 -> Subsystem6/6(vx2)  "<vx>"
  Bus Selector9/4 -> Subsystem6/4(xx5)  "<xx>"
  [state] -> Bus Selector5/1
  Subsystem2/1(utx) -> Subsystem8/2(utz)
  Bus Selector5/1 -> Subsystem8/1(vz4)  "<vz>"
  [state] -> Bus Selector4/1
  [gain] -> Subsystem8/3(gain)
  Bus Selector6/3 -> Subsystem12/6(vz)  "<vz>"
  Bus Selector6/1 -> Subsystem12/4(vx)  "<vx>"
  [Sx] -> Subsystem12/1(Sx)
  [Sz] -> Subsystem12/3(Sz)
  Subsystem12/1(" gain") -> [gain]
  Subsystem6/1(utx) -> Subsystem4/2(utx)
  In19/1 -> Bus Selector10/1, Bus Selector9/1, Bus Selector11/1, [state]
  [state] -> Bus Selector6/1
  Bus Selector4/1 -> Subsystem7/1(vy4)  "<vy>"
  Subsystem1/1(utx) -> Subsystem7/2(uty)
  Bus Selector3/1 -> Subsystem4/1(vx4)  "<vx>"
  Subsystem7/2(Sy) -> [Sy]
  [gain] -> Subsystem7/3(gain)
  [Sy] -> Subsystem12/2(Sy)
  [gain] -> Subsystem4/3(gain)
  [state] -> Bus Selector3/1
  Subsystem8/2(Sz) -> [Sz]
  Bus Selector6/2 -> Subsystem12/5(vy)  "<vy>"
  Subsystem4/2(Sx) -> [Sx]
  Subsystem3/1(udtx) -> Bus Creator/1  "ux"
  Subsystem3/2(udty) -> Bus Creator/2  "uy"
  Subsystem3/3(udtz) -> Bus Creator/3  "uz"
  Subsystem4/1(ux) -> Subsystem3/1(utx)
  Subsystem7/1(ux) -> Subsystem3/5(uty)
  Subsystem8/1(ux) -> Subsystem3/9(utz)
  [state] -> Bus Selector7/1
  Bus Selector8/1 -> Subsystem3/6(ux)  "<ux>"
  Bus Selector7/2 -> Subsystem3/3(vy)  "<vy>"
  Bus Selector8/2 -> Subsystem3/7(uy)  "<uy>"
  [state] -> Bus Selector8/1
  Bus Selector7/1 -> Subsystem3/2(vx)  "<vx>"
  Bus Selector7/3 -> Subsystem3/4(vz)  "<vz>"
  Bus Selector8/3 -> Subsystem3/8(uz)  "<uz>"

== system chap04_46/Subsystem/Subsystem4 ==
  In19 : Inport
  Bus Creator : BusCreator  Inputs=3
  Bus Selector : BusSelector  OutputSignals=state(t).node6.xx,state(t).node0.xx,state(t).node1.xx,state(t).node2.xx,state(t).node6.vx,state(t).node0.vx,state(t).node1.vx,state(t).node2.vx
  Bus Selector1 : BusSelector  OutputSignals=state(t).node6.xy,state(t).node0.xy,state(t).node1.xy,state(t).node2.xy,state(t).node6.vy,state(t).node0.vy,state(t).node1.vy,state(t).node2.vy
  Bus Selector2 : BusSelector  OutputSignals=state(t).node6.xz,state(t).node0.xz,state(t).node1.xz,state(t).node2.xz,state(t).node6.vz,state(t).node0.vz,state(t).node1.vz,state(t).node2.vz
  Bus Selector3 : BusSelector  OutputSignals=state(t).node6.vx,state(t).node0.vx
  Bus Selector4 : BusSelector  OutputSignals=state(t).node6.vy,state(t).node0.vx
  Bus Selector5 : BusSelector  OutputSignals=state(t).node6.vz,state(t).node0.vz
  Bus Selector6 : BusSelector  OutputSignals=state(t).node6.vx,state(t).node6.vy,state(t).node6.vz
  Bus Selector7 : BusSelector  OutputSignals=state(t).node6.vx,state(t).node6.vy,state(t).node6.vz
  Bus Selector8 : BusSelector  OutputSignals=control.node6.ux,control.node6.uy,control.node6.uz
  Subsystem1 : Subsystem
  Subsystem12 : Subsystem
  Subsystem2 : Subsystem
  Subsystem3 : Subsystem
  Subsystem4 : Subsystem
      settings: PortSchema="{\"entries\":[{\"content\":{\"sides\":[{\"content\":{\"connectorIds\":[\"In1\",\"In2\",\"In3\",\"In4\"]},\"type\":\"ConnectorPlacement.EquallySpacedRectSide\",\"uuid\":\"3c32f130-2df4-4697-80e9-267a8217898e\"},{\"content\":{\"connectorIds\":[\"Out1\"],\"side\":\"RIGHT\"},\"type\":\"ConnectorPlacement.EquallySpacedRectSide\",\"uuid\":\"840675a7-4714-440f-a6ce-75eff1b2763f\"},{\"content\":{\"connectorIds\":[],\"side\":\"TOP\"},\"type\":\"ConnectorPlacement.EquallySpacedRectSide\",\"uuid\":\"5c23af56-4ec3-4a39-a531-12998a0be3c8\"},{\"content\":{\"connectorIds\":[\"Out2\"],\"side\":\"BOTTOM\"},\"type\":\"ConnectorPlacement.EquallySpacedRectSide\",\"uuid\":\"31d953fb-65a0-42e9-a844-060de010f298\"}]},\"type\":\"ConnectorPlacement.EquallySpacedConnector\",\"uuid\":\"61b27aa3-5880-401e-bae3-4611093a191a\"}],\"packageUris\":[\"http://schema.mathworks.com/mf0/Connector/R2020b\"],\"version\":\"1.0\"}"
  Subsystem6 : Subsystem
  Subsystem7 : Subsystem
      settings: PortSchema="{\"entries\":[{\"content\":{\"sides\":[{\"content\":{\"connectorIds\":[\"In1\",\"In2\",\"In3\",\"In4\"]},\"type\":\"ConnectorPlacement.EquallySpacedRectSide\",\"uuid\":\"3c32f130-2df4-4697-80e9-267a8217898e\"},{\"content\":{\"connectorIds\":[\"Out1\"],\"side\":\"RIGHT\"},\"type\":\"ConnectorPlacement.EquallySpacedRectSide\",\"uuid\":\"840675a7-4714-440f-a6ce-75eff1b2763f\"},{\"content\":{\"connectorIds\":[],\"side\":\"TOP\"},\"type\":\"ConnectorPlacement.EquallySpacedRectSide\",\"uuid\":\"5c23af56-4ec3-4a39-a531-12998a0be3c8\"},{\"content\":{\"connectorIds\":[\"Out2\"],\"side\":\"BOTTOM\"},\"type\":\"ConnectorPlacement.EquallySpacedRectSide\",\"uuid\":\"31d953fb-65a0-42e9-a844-060de010f298\"}]},\"type\":\"ConnectorPlacement.EquallySpacedConnector\",\"uuid\":\"61b27aa3-5880-401e-bae3-4611093a191a\"}],\"packageUris\":[\"http://schema.mathworks.com/mf0/Connector/R2020b\"],\"version\":\"1.0\"}"
  Subsystem8 : Subsystem
      settings: PortSchema="{\"entries\":[{\"content\":{\"sides\":[{\"content\":{\"connectorIds\":[\"In1\",\"In2\",\"In3\",\"In4\"]},\"type\":\"ConnectorPlacement.EquallySpacedRectSide\",\"uuid\":\"3c32f130-2df4-4697-80e9-267a8217898e\"},{\"content\":{\"connectorIds\":[\"Out1\"],\"side\":\"RIGHT\"},\"type\":\"ConnectorPlacement.EquallySpacedRectSide\",\"uuid\":\"840675a7-4714-440f-a6ce-75eff1b2763f\"},{\"content\":{\"connectorIds\":[],\"side\":\"TOP\"},\"type\":\"ConnectorPlacement.EquallySpacedRectSide\",\"uuid\":\"5c23af56-4ec3-4a39-a531-12998a0be3c8\"},{\"content\":{\"connectorIds\":[\"Out2\"],\"side\":\"BOTTOM\"},\"type\":\"ConnectorPlacement.EquallySpacedRectSide\",\"uuid\":\"31d953fb-65a0-42e9-a844-060de010f298\"}]},\"type\":\"ConnectorPlacement.EquallySpacedConnector\",\"uuid\":\"61b27aa3-5880-401e-bae3-4611093a191a\"}],\"packageUris\":[\"http://schema.mathworks.com/mf0/Connector/R2020b\"],\"version\":\"1.0\"}"
  u6 : Outport
  wires:
  Bus Creator/1 -> u6/1  "node6"
  Bus Selector/1 -> Subsystem6/1(xx6)  "<xx>"
  Bus Selector/3 -> Subsystem6/3(xx1)  "<xx>"
  Bus Selector/4 -> Subsystem6/4(xx2)  "<xx>"
  Bus Selector6/3 -> Subsystem12/6(vz)  "<vz>"
  Bus Selector6/1 -> Subsystem12/4(vx)  "<vx>"
  [Sx] -> Subsystem12/1(Sx)
  [Sz] -> Subsystem12/3(Sz)
  Subsystem12/1(" gain") -> [gain]
  In19/1 -> Bus Selector1/1, Bus Selector/1, Bus Selector2/1, [state]
  [state] -> Bus Selector6/1
  [Sy] -> Subsystem12/2(Sy)
  Bus Selector6/2 -> Subsystem12/5(vy)  "<vy>"
  Subsystem3/3(udtz) -> Bus Creator/3  "uz"
  Subsystem3/2(udty) -> Bus Creator/2  "uy"
  Subsystem3/1(udtx) -> Bus Creator/1  "ux"
  Bus Selector7/3 -> Subsystem3/4(vz)  "<vz>"
  Bus Selector7/1 -> Subsystem3/2(vx)  "<vx>"
  [state] -> Bus Selector8/1
  Bus Selector8/1 -> Subsystem3/6(ux)  "<ux>"
  Bus Selector8/2 -> Subsystem3/7(uy)  "<uy>"
  Bus Selector7/2 -> Subsystem3/3(vy)  "<vy>"
  [state] -> Bus Selector7/1
  Bus Selector8/3 -> Subsystem3/8(uz)  "<uz>"
  Bus Selector/2 -> Subsystem6/2(xx0)  "<xx>"
  Bus Selector/5 -> Subsystem6/5(vx6)  "<vx>"
  Bus Selector/6 -> Subsystem6/6(vx0)  "<vx>"
  Bus Selector/7 -> Subsystem6/7(vx1)  "<vx>"
  Bus Selector/8 -> Subsystem6/8(vx2)  "<vx>"
  Bus Selector1/1 -> Subsystem1/1(xx6)  "<xy>"
  Bus Selector1/2 -> Subsystem1/2(xx0)  "<xy>"
  Bus Selector1/3 -> Subsystem1/3(xx1)  "<xy>"
  Bus Selector1/4 -> Subsystem1/4(xx2)  "<xy>"
  Bus Selector1/5 -> Subsystem1/5(vx6)  "<vy>"
  Bus Selector1/6 -> Subsystem1/6(vx0)  "<vy>"
  Bus Selector1/7 -> Subsystem1/7(vx1)  "<vy>"
  Bus Selector1/8 -> Subsystem1/8(vx2)  "<vy>"
  Bus Selector2/1 -> Subsystem2/1(xx6)  "<xz>"
  Bus Selector2/2 -> Subsystem2/2(xx0)  "<xz>"
  Bus Selector2/3 -> Subsystem2/3(xx1)  "<xz>"
  Bus Selector2/4 -> Subsystem2/4(xx2)  "<xz>"
  Bus Selector2/5 -> Subsystem2/5(vx6)  "<vz>"
  Bus Selector2/6 -> Subsystem2/6(vx0)  "<vz>"
  Bus Selector2/7 -> Subsystem2/7(vx1)  "<vz>"
  Bus Selector2/8 -> Subsystem2/8(vx2)  "<vz>"
  Subsystem4/2(Sx) -> [Sx]
  Bus Selector5/2 -> Subsystem8/2(vz0)  "<vz>"
  Subsystem7/2(Sy) -> [Sy]
  Subsystem8/2(Sz) -> [Sz]
  [gain] -> Subsystem7/4(gain)
  Subsystem1/1(utx) -> Subsystem7/3(uty)
  Subsystem2/1(utx) -> Subsystem8/3(utz)
  [state] -> Bus Selector3/1
  Bus Selector5/1 -> Subsystem8/1(vz6)  "<vz>"
  Bus Selector4/2 -> Subsystem7/2(vy0)  "<vx>"
  [gain] -> Subsystem4/4(gain)
  [state] -> Bus Selector5/1
  Subsystem8/1(ux) -> Subsystem3/9(utz)
  Subsystem6/1(utx) -> Subsystem4/3(utx)
  Subsystem7/1(ux) -> Subsystem3/5(uty)
  Subsystem4/1(ux) -> Subsystem3/1(utx)
  Bus Selector3/1 -> Subsystem4/1(vx6)  "<vx>"
  Bus Selector3/2 -> Subsystem4/2(vx0)  "<vx>"
  [gain] -> Subsystem8/4(gain)
  [state] -> Bus Selector4/1
  Bus Selector4/1 -> Subsystem7/1(vy6)  "<vy>"

== system chap04_46/Subsystem/Subsystem5 ==
  In19 : Inport
  Bus Creator : BusCreator  Inputs=3
  Bus Selector10 : BusSelector  OutputSignals=state(t).node3.xy,state(t).node1.xy,state(t).node4.xy,state(t).node5.xy,state(t).node3.vy,state(t).node1.vy,state(t).node4.vy,state(t).node5.vy
  Bus Selector11 : BusSelector  OutputSignals=state(t).node3.xz,state(t).node1.xz,state(t).node4.xz,state(t).node5.xz,state(t).node3.vz,state(t).node1.vz,state(t).node4.vz,state(t).node5.vz
  Bus Selector3 : BusSelector  OutputSignals=state(t).node3.vx
  Bus Selector4 : BusSelector  OutputSignals=state(t).node3.vy
  Bus Selector5 : BusSelector  OutputSignals=state(t).node3.vz
  Bus Selector6 : BusSelector  OutputSignals=state(t).node3.vx,state(t).node3.vy,state(t).node3.vz
  Bus Selector7 : BusSelector  OutputSignals=state(t).node3.vx,state(t).node3.vy,state(t).node3.vz
  Bus Selector8 : BusSelector  OutputSignals=control.node3.ux,control.node3.uy,control.node3.uz
  Bus Selector9 : BusSelector  OutputSignals=state(t).node3.xx,state(t).node1.xx,state(t).node4.xx,state(t).node5.xx,state(t).node3.vx,state(t).node1.vx,state(t).node4.vx,state(t).node5.vx
  Subsystem1 : Subsystem
  Subsystem12 : Subsystem
  Subsystem2 : Subsystem
  Subsystem3 : Subsystem
  Subsystem4 : Subsystem
      settings: PortSchema="{\"entries\":[{\"content\":{\"sides\":[{\"content\":{\"connectorIds\":[\"In1\",\"In2\",\"In3\"]},\"type\":\"ConnectorPlacement.EquallySpacedRectSide\",\"uuid\":\"3c32f130-2df4-4697-80e9-267a8217898e\"},{\"content\":{\"connectorIds\":[\"Out1\"],\"side\":\"RIGHT\"},\"type\":\"ConnectorPlacement.EquallySpacedRectSide\",\"uuid\":\"840675a7-4714-440f-a6ce-75eff1b2763f\"},{\"content\":{\"connectorIds\":[],\"side\":\"TOP\"},\"type\":\"ConnectorPlacement.EquallySpacedRectSide\",\"uuid\":\"5c23af56-4ec3-4a39-a531-12998a0be3c8\"},{\"content\":{\"connectorIds\":[\"Out2\"],\"side\":\"BOTTOM\"},\"type\":\"ConnectorPlacement.EquallySpacedRectSide\",\"uuid\":\"31d953fb-65a0-42e9-a844-060de010f298\"}]},\"type\":\"ConnectorPlacement.EquallySpacedConnector\",\"uuid\":\"61b27aa3-5880-401e-bae3-4611093a191a\"}],\"packageUris\":[\"http://schema.mathworks.com/mf0/Connector/R2020b\"],\"version\":\"1.0\"}"
  Subsystem6 : Subsystem
  Subsystem7 : Subsystem
      settings: PortSchema="{\"entries\":[{\"content\":{\"sides\":[{\"content\":{\"connectorIds\":[\"In1\",\"In2\",\"In3\"]},\"type\":\"ConnectorPlacement.EquallySpacedRectSide\",\"uuid\":\"3c32f130-2df4-4697-80e9-267a8217898e\"},{\"content\":{\"connectorIds\":[\"Out1\"],\"side\":\"RIGHT\"},\"type\":\"ConnectorPlacement.EquallySpacedRectSide\",\"uuid\":\"840675a7-4714-440f-a6ce-75eff1b2763f\"},{\"content\":{\"connectorIds\":[],\"side\":\"TOP\"},\"type\":\"ConnectorPlacement.EquallySpacedRectSide\",\"uuid\":\"5c23af56-4ec3-4a39-a531-12998a0be3c8\"},{\"content\":{\"connectorIds\":[\"Out2\"],\"side\":\"BOTTOM\"},\"type\":\"ConnectorPlacement.EquallySpacedRectSide\",\"uuid\":\"31d953fb-65a0-42e9-a844-060de010f298\"}]},\"type\":\"ConnectorPlacement.EquallySpacedConnector\",\"uuid\":\"61b27aa3-5880-401e-bae3-4611093a191a\"}],\"packageUris\":[\"http://schema.mathworks.com/mf0/Connector/R2020b\"],\"version\":\"1.0\"}"
  Subsystem8 : Subsystem
      settings: PortSchema="{\"entries\":[{\"content\":{\"sides\":[{\"content\":{\"connectorIds\":[\"In1\",\"In2\",\"In3\"]},\"type\":\"ConnectorPlacement.EquallySpacedRectSide\",\"uuid\":\"3c32f130-2df4-4697-80e9-267a8217898e\"},{\"content\":{\"connectorIds\":[\"Out1\"],\"side\":\"RIGHT\"},\"type\":\"ConnectorPlacement.EquallySpacedRectSide\",\"uuid\":\"840675a7-4714-440f-a6ce-75eff1b2763f\"},{\"content\":{\"connectorIds\":[],\"side\":\"TOP\"},\"type\":\"ConnectorPlacement.EquallySpacedRectSide\",\"uuid\":\"5c23af56-4ec3-4a39-a531-12998a0be3c8\"},{\"content\":{\"connectorIds\":[\"Out2\"],\"side\":\"BOTTOM\"},\"type\":\"ConnectorPlacement.EquallySpacedRectSide\",\"uuid\":\"31d953fb-65a0-42e9-a844-060de010f298\"}]},\"type\":\"ConnectorPlacement.EquallySpacedConnector\",\"uuid\":\"61b27aa3-5880-401e-bae3-4611093a191a\"}],\"packageUris\":[\"http://schema.mathworks.com/mf0/Connector/R2020b\"],\"version\":\"1.0\"}"
  u3 : Outport
  wires:
  Bus Creator/1 -> u3/1  "node3"
  [state] -> Bus Selector6/1
  [Sz] -> Subsystem12/3(Sz)
  [Sx] -> Subsystem12/1(Sx)
  Bus Selector6/3 -> Subsystem12/6(vz)  "<vz>"
  [Sy] -> Subsystem12/2(Sy)
  Bus Selector6/1 -> Subsystem12/4(vx)  "<vx>"
  Bus Selector6/2 -> Subsystem12/5(vy)  "<vy>"
  Subsystem3/1(udtx) -> Bus Creator/1  "ux"
  Subsystem3/2(udty) -> Bus Creator/2  "uy"
  Subsystem3/3(udtz) -> Bus Creator/3  "uz"
  [state] -> Bus Selector7/1
  Bus Selector8/1 -> Subsystem3/6(ux)  "<ux>"
  Bus Selector7/2 -> Subsystem3/3(vy)  "<vy>"
  Bus Selector8/2 -> Subsystem3/7(uy)  "<uy>"
  [state] -> Bus Selector8/1
  Bus Selector7/1 -> Subsystem3/2(vx)  "<vx>"
  Bus Selector7/3 -> Subsystem3/4(vz)  "<vz>"
  Bus Selector8/3 -> Subsystem3/8(uz)  "<uz>"
  Subsystem12/1(" gain") -> [gain]
  Bus Selector11/8 -> Subsystem2/8(vz5)  "<vz>"
  In19/1 -> Bus Selector9/1, Bus Selector10/1, Bus Selector11/1, [state]
  Bus Selector10/4 -> Subsystem1/4(xy5)  "<xy>"
  Bus Selector9/4 -> Subsystem6/4(xx5)  "<xx>"
  Bus Selector9/2 -> Subsystem6/2(xx1)  "<xx>"
  Bus Selector9/1 -> Subsystem6/1(xx3)  "<xx>"
  Bus Selector9/8 -> Subsystem6/8(vx5)  "<vx>"
  Bus Selector11/7 -> Subsystem2/7(vz4)  "<vz>"
  Bus Selector10/5 -> Subsystem1/5(vy3)  "<vy>"
  Bus Selector10/1 -> Subsystem1/1(xy3)  "<xy>"
  Bus Selector9/3 -> Subsystem6/3(xx4)  "<xx>"
  Bus Selector9/5 -> Subsystem6/5(vx3)  "<vx>"
  Bus Selector10/6 -> Subsystem1/6(vy1)  "<vy>"
  Bus Selector11/3 -> Subsystem2/3(xz4)  "<xz>"
  Bus Selector10/8 -> Subsystem1/8(vy5)  "<vy>"
  Bus Selector11/1 -> Subsystem2/1(xz3)  "<xz>"
  Bus Selector10/3 -> Subsystem1/3(xy4)  "<xy>"
  Bus Selector10/2 -> Subsystem1/2(xy1)  "<xy>"
  Bus Selector10/7 -> Subsystem1/7(vy4)  "<vy>"
  Bus Selector11/2 -> Subsystem2/2(xz1)  "<xz>"
  Bus Selector11/4 -> Subsystem2/4(xz5)  "<xz>"
  Bus Selector11/6 -> Subsystem2/6(vz1)  "<vz>"
  Bus Selector11/5 -> Subsystem2/5(vz3)  "<vz>"
  Bus Selector9/7 -> Subsystem6/7(vx4)  "<vx>"
  Bus Selector9/6 -> Subsystem6/6(vx1)  "<vx>"
  Subsystem6/1(p3x) -> Subsystem4/2(utx)
  [gain] -> Subsystem7/3(gain)
  Bus Selector4/1 -> Subsystem7/1(vy3)  "<vy>"
  [state] -> Bus Selector5/1
  [state] -> Bus Selector3/1
  Subsystem4/2(Sx) -> [Sx]
  Bus Selector3/1 -> Subsystem4/1(vx3)  "<vx>"
  Subsystem7/1(ux) -> Subsystem3/5(uty)
  Bus Selector5/1 -> Subsystem8/1(vz3)  "<vz>"
  [gain] -> Subsystem4/3(gain)
  Subsystem8/1(ux) -> Subsystem3/9(utz)
  [gain] -> Subsystem8/3(gain)
  Subsystem2/1(p3z) -> Subsystem8/2(utz)
  Subsystem4/1(ux) -> Subsystem3/1(utx)
  Subsystem1/1(p3y) -> Subsystem7/2(uty)
  [state] -> Bus Selector4/1
  Subsystem8/2(Sz) -> [Sz]
  Subsystem7/2(Sy) -> [Sy]

== system chap04_46/Subsystem1/Subsystem ==
  dx : Inport
  dy : Inport  Port=2
  dz : Inport  Port=3
  ut1x : Inport  Port=4
  ut1y : Inport  Port=5
  ut1z : Inport  Port=6
  Add : Sum
  Add1 : Sum
  Add2 : Sum
  Add3 : Sum  Inputs=-+
  Add4 : Sum  Inputs=-+
  Add5 : Sum  Inputs=-+
  Bus Creator1 : BusCreator  Inputs=6
  Constant : Constant  Value=-1
  Constant1 : Constant
  Constant2 : Constant  Value=0
  Discrete-Time Integrator{,15..17} (4 alike) : DiscreteIntegrator  SampleTime=-1  ICPrevOutput=DiscIntNeverNeededParam  ICPrevScaledInput=DiscIntNeverNeededParam
  Discrete-Time Integrator14 : DiscreteIntegrator  InitialCondition=-1  SampleTime=-1  ICPrevOutput=DiscIntNeverNeededParam  ICPrevScaledInput=DiscIntNeverNeededParam
  Discrete-Time Integrator5 : DiscreteIntegrator  InitialCondition=1  SampleTime=-1  ICPrevOutput=DiscIntNeverNeededParam  ICPrevScaledInput=DiscIntNeverNeededParam
  node1 : Outport
  wires:
  ut1y/1 -> Add1/2
  ut1z/1 -> Add2/2
  Discrete-Time Integrator17/1 -> Discrete-Time Integrator15/1, Bus Creator1/5  "vy"
  Discrete-Time Integrator/1 -> Discrete-Time Integrator5/1, Bus Creator1/6  "vz"
  ut1x/1 -> Add/2
  Discrete-Time Integrator16/1 -> Bus Creator1/4, Discrete-Time Integrator14/1  "vx"
  Bus Creator1/1 -> node1/1  "node1"
  Add5/1 -> Bus Creator1/3  "xz"
  Add4/1 -> Bus Creator1/2  "xy"
  Add3/1 -> Bus Creator1/1  "xx"
  Add/1 -> Discrete-Time Integrator16/1
  Add1/1 -> Discrete-Time Integrator17/1
  Add2/1 -> Discrete-Time Integrator/1
  dy/1 -> Add1/1
  dz/1 -> Add2/1
  dx/1 -> Add/1
  Discrete-Time Integrator14/1 -> Add3/2
  Discrete-Time Integrator5/1 -> Add5/2
  Discrete-Time Integrator15/1 -> Add4/2
  Constant/1 -> Add3/1
  Constant1/1 -> Add4/1
  Constant2/1 -> Add5/1

== system chap04_46/Subsystem1/Subsystem1 ==
  dx : Inport
  dy : Inport  Port=2
  dz : Inport  Port=3
  ut2x : Inport  Port=4
  ut2y : Inport  Port=5
  ut2z : Inport  Port=6
  Add : Sum
  Add1 : Sum
  Add2 : Sum
  Add3 : Sum  Inputs=-+
  Add4 : Sum  Inputs=-+
  Add5 : Sum  Inputs=-+
  Bus Creator1 : BusCreator  Inputs=6
  Constant : Constant
  Constant1 : Constant
  Constant2 : Constant  Value=0
  Discrete-Time Integrator : DiscreteIntegrator  SampleTime=-1  ICPrevOutput=DiscIntNeverNeededParam  ICPrevScaledInput=DiscIntNeverNeededParam
  Discrete-Time Integrator14 : DiscreteIntegrator  InitialCondition=1.5  SampleTime=-1  ICPrevOutput=DiscIntNeverNeededParam  ICPrevScaledInput=DiscIntNeverNeededParam
  Discrete-Time Integrator15 : DiscreteIntegrator  InitialCondition=0.5  SampleTime=-1  ICPrevOutput=DiscIntNeverNeededParam  ICPrevScaledInput=DiscIntNeverNeededParam
  Discrete-Time Integrator16 : DiscreteIntegrator  SampleTime=-1  ICPrevOutput=DiscIntNeverNeededParam  ICPrevScaledInput=DiscIntNeverNeededParam
  Discrete-Time Integrator17 : DiscreteIntegrator  SampleTime=-1  ICPrevOutput=DiscIntNeverNeededParam  ICPrevScaledInput=DiscIntNeverNeededParam
  Discrete-Time Integrator5 : DiscreteIntegrator  InitialCondition=1  SampleTime=-1  ICPrevOutput=DiscIntNeverNeededParam  ICPrevScaledInput=DiscIntNeverNeededParam
  node2 : Outport
  wires:
  Bus Creator1/1 -> node2/1  "node2"
  Discrete-Time Integrator16/1 -> Bus Creator1/4, Discrete-Time Integrator14/1  "vx"
  Discrete-Time Integrator/1 -> Discrete-Time Integrator5/1, Bus Creator1/6  "vz"
  Discrete-Time Integrator17/1 -> Bus Creator1/5, Discrete-Time Integrator15/1  "vy"
  dx/1 -> Add/1
  dy/1 -> Add1/1
  dz/1 -> Add2/1
  Add2/1 -> Discrete-Time Integrator/1
  Add1/1 -> Discrete-Time Integrator17/1
  Add/1 -> Discrete-Time Integrator16/1
  ut2x/1 -> Add/2
  ut2y/1 -> Add1/2
  ut2z/1 -> Add2/2
  Constant2/1 -> Add5/1
  Constant1/1 -> Add4/1
  Discrete-Time Integrator14/1 -> Add3/2
  Discrete-Time Integrator15/1 -> Add4/2
  Discrete-Time Integrator5/1 -> Add5/2
  Constant/1 -> Add3/1
  Add3/1 -> Bus Creator1/1  "xx"
  Add4/1 -> Bus Creator1/2  "xy"
  Add5/1 -> Bus Creator1/3  "xz"
